simulink model "diffworm"  (Simulink 7.9)
settings: Solver=ode3  StartTime=0.0  StopTime=100  FixedStep=0.02  RelTol=1e-3
settings Model: Creator=jamil  LastModifiedBy=jamil
settings DataIOCC: LimitDataPoints=off

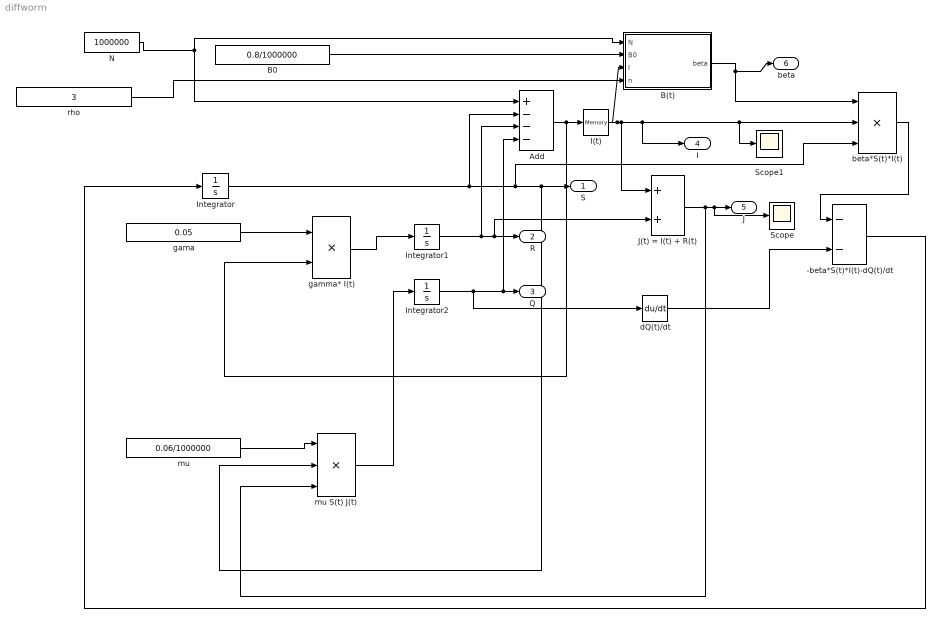
== system diffworm ==
  -beta*S(t)*I(t)-dQ(t)/dt : Sum  Inputs=--
  Add : Sum  Inputs=+---
  B(t) : Subsystem  TreatAsAtomicUnit=on
  B0 : Constant  Value=0.8/1000000
  I(t) : Memory  X0=1
  Integrator : Integrator  InitialCondition=1000000-1
  Integrator1 : Integrator
  Integrator2 : Integrator
  J(t) = I(t) + R(t) : Sum
  N : Constant  Value=1000000
  Scope : Scope
  Scope1 : Scope
  beta*S(t)*I(t) : Product  Inputs=3  RndMeth=Zero
  dQ(t)/dt : Derivative
  gama : Constant  Value=0.05
  gamma* I(t) : Product  RndMeth=Zero
  mu : Constant  Value=0.06/1000000
  mu S(t) J(t) : Product  Inputs=3  RndMeth=Zero
  rho : Constant  Value=3
  S : Outport
  R : Outport  Port=2
  Q : Outport  Port=3
  I : Outport  Port=4
  J : Outport  Port=5
  beta : Outport  Port=6
  wires:
  Integrator/1 -> Add/2, S/1, mu S(t) J(t)/2, beta*S(t)*I(t)/3
  Integrator1/1 -> Add/3, R/1, J(t) = I(t) + R(t)/2
  Integrator2/1 -> Q/1, Add/4, dQ(t)/dt/1
  N/1 -> B(t)/1(N), Add/1
  B0/1 -> B(t)/2(B0)
  rho/1 -> B(t)/4(n)
  Add/1 -> I(t)/1, gamma* I(t)/2
  J(t) = I(t) + R(t)/1 -> mu S(t) J(t)/3, J/1, Scope/1
  B(t)/1(beta) -> beta*S(t)*I(t)/1, beta/1
  beta*S(t)*I(t)/1 -> -beta*S(t)*I(t)-dQ(t)/dt/1
  dQ(t)/dt/1 -> -beta*S(t)*I(t)-dQ(t)/dt/2
  I(t)/1 -> J(t) = I(t) + R(t)/1, I/1, beta*S(t)*I(t)/2, Scope1/1, B(t)/3(I)
  gama/1 -> gamma* I(t)/1
  -beta*S(t)*I(t)-dQ(t)/dt/1 -> Integrator/1
  gamma* I(t)/1 -> Integrator1/1
  mu/1 -> mu S(t) J(t)/1
  mu S(t) J(t)/1 -> Integrator2/1

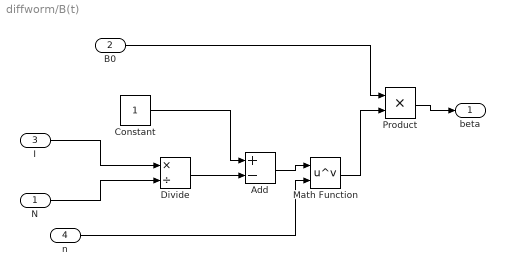
== system diffworm/B(t) ==
  N : Inport
  B0 : Inport  Port=2
  I : Inport  Port=3
  n : Inport  Port=4
  Add : Sum  Inputs=+-
  Constant : Constant
  Divide : Product  Inputs=*/
  Math Function : Math  Operator=pow  SaturateOnIntegerOverflow=on
  Product : Product  RndMeth=Zero
  beta : Outport
  wires:
  B0/1 -> Product/1
  I/1 -> Divide/1
  N/1 -> Divide/2
  Divide/1 -> Add/2
  Constant/1 -> Add/1
  Add/1 -> Math Function/1
  Product/1 -> beta/1
  Math Function/1 -> Product/2
  n/1 -> Math Function/2
